simulink model "gm_uz_pmsm_model_9ph"  (R2021b)
settings: Solver=FixedStepAuto  StartTime=0.0  StopTime=0.8  RelTol=1e-3
PreLoadFcn:
  | uz_pmsm_model_9ph_init_parameter
undefined symbols (not defined in the file or in its folder): a, b, c, friction_coefficient, inertia, k_i_d, k_i_q, k_p_d, k_p_q, Kpd, L_d, L_o1, L_o2, L_q, L_x1, L_x2, L_y1, L_y2, L_zero, polepair, psi_pm, R_1, static_friction_torque, Tnd
libraries: hdlmdlgenlib x190, hdlsllib x90, dspsigops x17, simulink x3, slpidlib x2, spsAlphaBetaZerotodq0Lib x1, pid_lib x1, spsdq0toAlphaBetaZeroLib x1
(part 1 of 6)
settings Model: Creator=ts  LastModifiedBy=valen
settings SolverCC: AlgebraicLoopSolver=TrustRegion  AutoInsertRateTranBlk=on
settings DataIOCC: LimitDataPoints=on  SaveOutput=off  SaveTime=off
settings OptimizationCC: BlockReduction=off  ConditionallyExecuteInputs=off  DefaultParameterBehavior=Inlined  LifeSpan=inf
settings DebuggingCC: AlgebraicLoopMsg=error  ArtificialAlgebraicLoopMsg=none  InheritedTsInSrcMsg=none  SingleTaskRateTransMsg=error  AllowSymbolicDim=off  StrictBusMsg=ErrorOnBusTreatedAsVector  SFUnexpectedBacktrackingDiag=warning  SFNoUnconditionalDefaultTransitionDiag=warning  SFExecutionAtInitializationDiag=none  SFMachineParentedDataDiag=warning  ArithmeticOperatorsInVariantConditions=warning
settings HardwareCC: ProdBitPerPointer=32  ProdBitPerSizeT=32  ProdBitPerPtrDiffT=32  ProdLargestAtomicFloat=None  ProdIntDivRoundTo=Undefined  ProdEndianess=Unspecified  ProdWordSize=32  ProdHWDeviceType=ASIC/FPGA->ASIC/FPGA  ProdEqTarget=off
settings SFSimCC: SimUseLocalCustomCode=off  CustomCodeUndefinedFunction=UseInterfaceOnly
settings RTWCC: RTWUseLocalCustomCode=off
settings CodeAppCC: StateflowObjectComments=on
settings GRTTargetCC: TargetLangStandard=C89/C90 (ANSI)
settings ConfigComp: CovScope=ReferencedModels  CovMetricSettings=dw  CovSaveCumulativeToWorkspaceVar=on  CovSaveSingleToWorkspaceVar=on  CovExternalEMLEnable=off  CovSFcnEnable=off

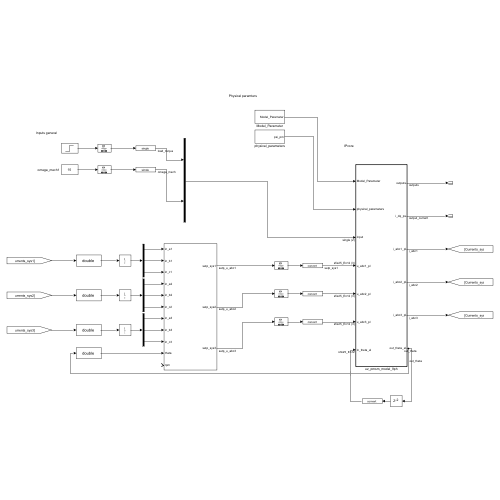
[thumbnail: Simulink's stored preview of the top-level diagram]
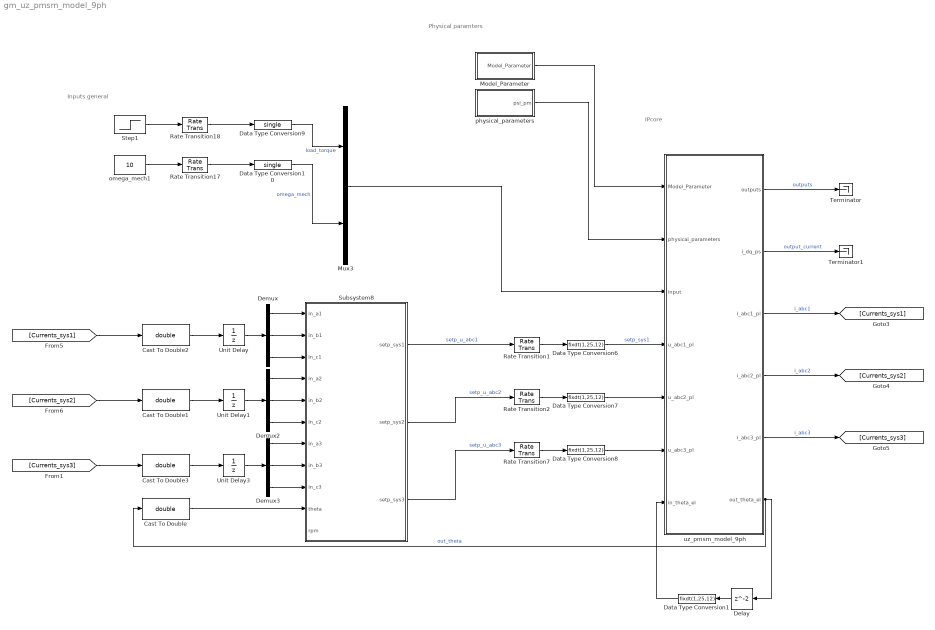
== system gm_uz_pmsm_model_9ph ==
  note: Inputs general
  note: Physical paramters
  note: IPcore
  Cast To Double{,1..3} (4 alike) : DataTypeConversion  OutDataTypeStr=double
  Data Type Conversion{1,6..8} (4 alike) : DataTypeConversion  OutDataTypeStr=fixdt(1,25,12)  RndMeth=Nearest
  Data Type Conversion10 : DataTypeConversion  OutDataTypeStr=single  RndMeth=Nearest
  Data Type Conversion9 : DataTypeConversion  OutDataTypeStr=single  RndMeth=Nearest
  Delay : Delay
  Demux : Demux  Outputs=3
  Demux2 : Demux  Outputs=3
  Demux3 : Demux  Outputs=3
  Model_Parameter : Subsystem
  Mux3 : Mux  Inputs=2
  Rate Transition{1..2,7,17..18} (5 alike) : RateTransition  OutPortSampleTime=ts
  Step1 : Step  Time=0.25  After=20  SampleTime=0
  Subsystem8 : Subsystem
  Terminator : Terminator
  Terminator1 : Terminator
  Unit Delay : UnitDelay  SampleTime=-1  HasFrameUpgradeWarning=on
  Unit Delay1 : UnitDelay  SampleTime=-1  HasFrameUpgradeWarning=on
  Unit Delay3 : UnitDelay  SampleTime=-1  HasFrameUpgradeWarning=on
  omega_mech1 : Constant  Value=10
  physical_parameters : Subsystem
  uz_pmsm_model_9ph : Subsystem  TreatAsAtomicUnit=on
  wires:
  Rate Transition7/1 -> Data Type Conversion8/1
  Rate Transition2/1 -> Data Type Conversion7/1
  Rate Transition1/1 -> Data Type Conversion6/1
  Cast To Double3/1 -> Unit Delay3/1
  Cast To Double2/1 -> Unit Delay/1
  Cast To Double1/1 -> Unit Delay1/1
  Cast To Double/1 -> Subsystem8/10(theta)
  Demux2/3 -> Subsystem8/6(in_c2)
  Demux2/2 -> Subsystem8/5(in_b2)
  Demux/1 -> Subsystem8/1(in_a1)
  Demux3/1 -> Subsystem8/7(in_a3)
  [Currents_sys3] -> Cast To Double3/1
  Unit Delay/1 -> Demux/1
  Demux3/3 -> Subsystem8/9(in_c3)
  [Currents_sys2] -> Cast To Double1/1
  [Currents_sys1] -> Cast To Double2/1
  Demux/3 -> Subsystem8/3(in_c1)
  Unit Delay1/1 -> Demux2/1
  Demux3/2 -> Subsystem8/8(in_b3)
  Demux2/1 -> Subsystem8/4(in_a2)
  Demux/2 -> Subsystem8/2(in_b1)
  Unit Delay3/1 -> Demux3/1
  Data Type Conversion7/1 -> uz_pmsm_model_9ph/5(u_abc2_pl)
  Data Type Conversion8/1 -> uz_pmsm_model_9ph/6(u_abc3_pl)
  Subsystem8/3(setp_sys3) -> Rate Transition7/1  "setp_u_abc3"
  Subsystem8/2(setp_sys2) -> Rate Transition2/1  "setp_u_abc2"
  Data Type Conversion6/1 -> uz_pmsm_model_9ph/4(u_abc1_pl)  "setp_sys1"
  Subsystem8/1(setp_sys1) -> Rate Transition1/1  "setp_u_abc1"
  Delay/1 -> Data Type Conversion1/1
  uz_pmsm_model_9ph/6(out_theta_el) -> Cast To Double/1, Delay/1  "out_theta"
  uz_pmsm_model_9ph/4(i_abc2_pl) -> [Currents_sys2]  "i_abc2"
  uz_pmsm_model_9ph/5(i_abc3_pl) -> [Currents_sys3]  "i_abc3"
  uz_pmsm_model_9ph/3(i_abc1_pl) -> [Currents_sys1]  "i_abc1"
  uz_pmsm_model_9ph/2(i_dq_ps) -> Terminator1/1  "output_current"
  Data Type Conversion1/1 -> uz_pmsm_model_9ph/7(in_theta_el)
  Mux3/1 -> uz_pmsm_model_9ph/3(input)
  Data Type Conversion9/1 -> Mux3/1  "load_torque"
  Rate Transition17/1 -> Data Type Conversion10/1
  Data Type Conversion10/1 -> Mux3/2  "omega_mech"
  Step1/1 -> Rate Transition18/1
  Rate Transition18/1 -> Data Type Conversion9/1
  omega_mech1/1 -> Rate Transition17/1
  Model_Parameter/1(Model_Parameter) -> uz_pmsm_model_9ph/1(Model_Parameter)
  uz_pmsm_model_9ph/1(outputs) -> Terminator/1  "outputs"
  physical_parameters/1(psi_pm) -> uz_pmsm_model_9ph/2(physical_parameters)

== system gm_uz_pmsm_model_9ph/Model_Parameter ==
  note: This flag determines if omega_mech is used as an input value or
      | if the mechanical system is simulated by the model
  Bus Creator : BusCreator  Inputs=4
  Constant3 : Constant  Value=0
  Data Type Conversion{3..4,9..10} (4 alike) : DataTypeConversion  OutDataTypeStr=boolean
  Rate Transition{6,8,17..18} (4 alike) : RateTransition  OutPortSampleTime=ts
  simulate_mechanical : Constant  Value=false
  simulate_mechanical1 : Constant  Value=false
  simulate_mechanical2 : Constant  Value=false
  Model_Parameter : Outport
  wires:
  Data Type Conversion3/1 -> Bus Creator/1  "reset_integrators"
  Bus Creator/1 -> Model_Parameter/1
  Data Type Conversion4/1 -> Bus Creator/2  "simulate_mechanical"
  Data Type Conversion9/1 -> Bus Creator/3  "switch_pspl"
  Data Type Conversion10/1 -> Bus Creator/4  "control_dq_abc"
  Rate Transition18/1 -> Data Type Conversion10/1
  Rate Transition17/1 -> Data Type Conversion9/1
  simulate_mechanical1/1 -> Rate Transition17/1
  Constant3/1 -> Rate Transition6/1
  Rate Transition6/1 -> Data Type Conversion3/1
  Rate Transition8/1 -> Data Type Conversion4/1
  simulate_mechanical/1 -> Rate Transition8/1
  simulate_mechanical2/1 -> Rate Transition18/1

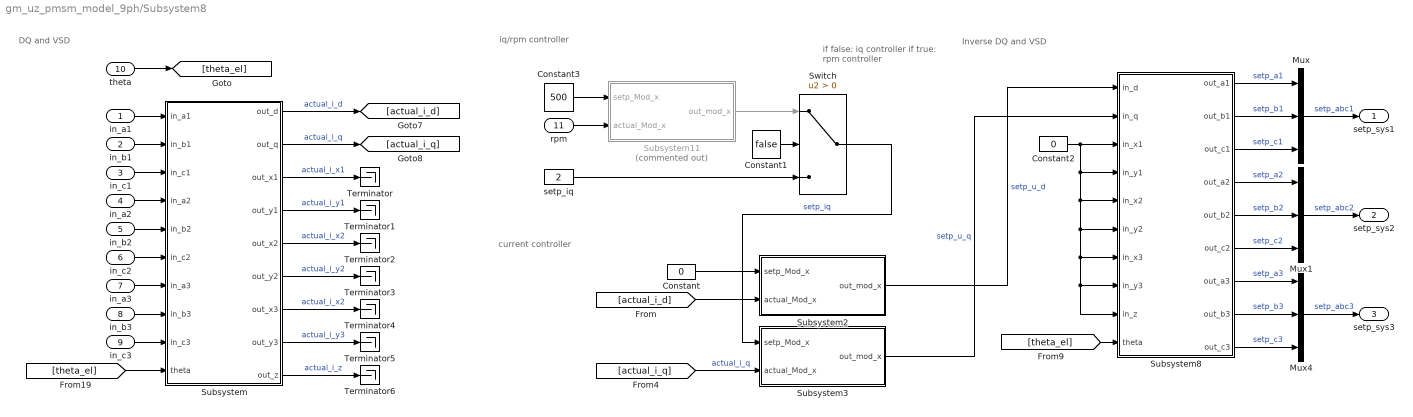
== system gm_uz_pmsm_model_9ph/Subsystem8 ==
  note: Inverse DQ and VSD
  note: if false: iq controller
      | if true: rpm controller
  note: iq/rpm controller
  note: current controller
  note: DQ and VSD
  in_a1 : Inport
  in_b1 : Inport  Port=2
  in_c1 : Inport  Port=3
  in_a2 : Inport  Port=4
  in_b2 : Inport  Port=5
  in_c2 : Inport  Port=6
  in_a3 : Inport  Port=7
  in_b3 : Inport  Port=8
  in_c3 : Inport  Port=9
  theta : Inport  Port=10
  rpm : Inport  Port=11
  Constant : Constant  Value=0
  Constant1 : Constant  Value=false
  Constant2 : Constant  Value=0
  Constant3 : Constant  Value=500
  Mux : Mux  Inputs=3
  Mux1 : Mux  Inputs=3
  Mux4 : Mux  Inputs=3
  Subsystem : Subsystem
  Subsystem11 : Subsystem  Commented=on
  Subsystem2 : Subsystem
  Subsystem3 : Subsystem
  Subsystem8 : Subsystem
  Switch : Switch  Criteria=u2 > Threshold
  Terminator{,1..6} (7 alike) : Terminator
  setp_iq : Constant  Value=2
  setp_sys1 : Outport
  setp_sys2 : Outport  Port=2
  setp_sys3 : Outport  Port=3
  wires:
  Subsystem2/1(out_mod_x) -> Subsystem8/1(in_d)  "setp_u_d"
  Subsystem3/1(out_mod_x) -> Subsystem8/2(in_q)  "setp_u_q"
  Constant3/1 -> Subsystem11/1(setp_Mod_x)
  setp_iq/1 -> Switch/3
  Constant1/1 -> Switch/2
  Switch/1 -> Subsystem3/1(setp_Mod_x)  "setp_iq"
  Subsystem11/1(out_mod_x) -> Switch/1
  Constant2/1 -> Subsystem8/4(in_y1), Subsystem8/5(in_x2), Subsystem8/6(in_y2), Subsystem8/7(in_x3), Subsystem8/9(in_z), Subsystem8/8(in_y3), Subsystem8/3(in_x1)
  [theta_el] -> Subsystem/10(theta)
  Subsystem/2(out_q) -> [actual_i_q]  "actual_i_q"
  Subsystem/1(out_d) -> [actual_i_d]  "actual_i_d"
  rpm/1 -> Subsystem11/2(actual_Mod_x)
  Subsystem8/9(out_c3) -> Mux4/3  "setp_c3"
  Subsystem8/8(out_b3) -> Mux4/2  "setp_b3"
  Subsystem8/7(out_a3) -> Mux4/1  "setp_a3"
  Mux4/1 -> setp_sys3/1  "setp_abc3"
  Subsystem8/4(out_a2) -> Mux1/1  "setp_a2"
  Subsystem8/5(out_b2) -> Mux1/2  "setp_b2"
  Subsystem8/6(out_c2) -> Mux1/3  "setp_c2"
  Mux1/1 -> setp_sys2/1  "setp_abc2"
  in_a3/1 -> Subsystem/7(in_a3)
  in_b3/1 -> Subsystem/8(in_b3)
  in_c3/1 -> Subsystem/9(in_c3)
  Subsystem/9(out_z) -> Terminator6/1  "actual_i_z"
  Subsystem/7(out_x3) -> Terminator4/1  "actual_i_x2"
  Subsystem/8(out_y3) -> Terminator5/1  "actual_i_y3"
  Mux/1 -> setp_sys1/1  "setp_abc1"
  theta/1 -> [theta_el]
  in_c2/1 -> Subsystem/6(in_c2)
  in_a2/1 -> Subsystem/4(in_a2)
  in_b2/1 -> Subsystem/5(in_b2)
  [actual_i_q] -> Subsystem3/2(actual_Mod_x)  "actual_i_q"
  in_a1/1 -> Subsystem/1(in_a1)
  Subsystem/5(out_x2) -> Terminator2/1  "actual_i_x2"
  Subsystem/6(out_y2) -> Terminator3/1  "actual_i_y2"
  Constant/1 -> Subsystem2/1(setp_Mod_x)
  [actual_i_d] -> Subsystem2/2(actual_Mod_x)
  in_c1/1 -> Subsystem/3(in_c1)
  Subsystem/3(out_x1) -> Terminator/1  "actual_i_x1"
  Subsystem8/3(out_c1) -> Mux/3  "setp_c1"
  Subsystem8/2(out_b1) -> Mux/2  "setp_b1"
  [theta_el] -> Subsystem8/10(theta)
  in_b1/1 -> Subsystem/2(in_b1)
  Subsystem8/1(out_a1) -> Mux/1  "setp_a1"
  Subsystem/4(out_y1) -> Terminator1/1  "actual_i_y1"

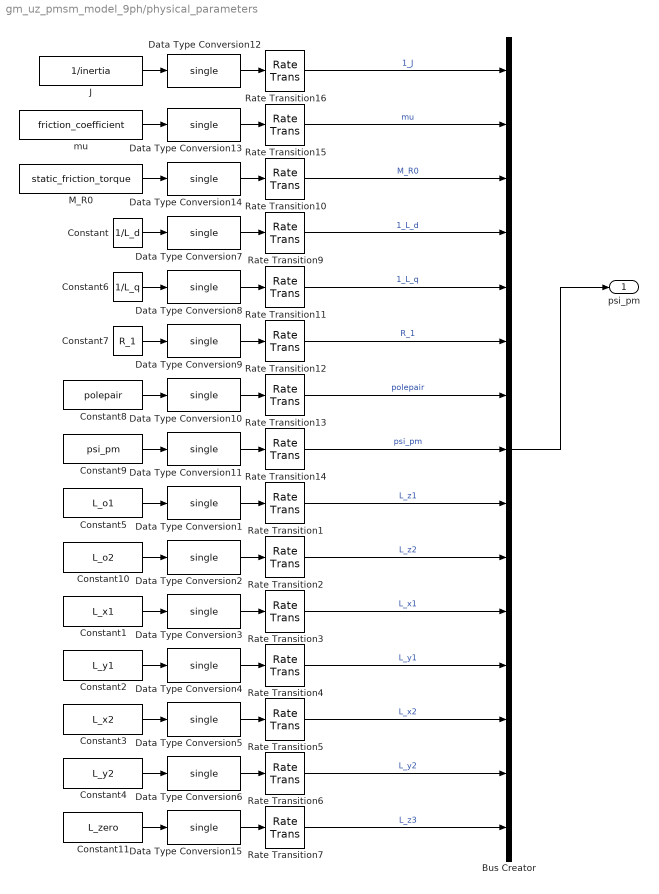
== system gm_uz_pmsm_model_9ph/physical_parameters ==
  Bus Creator : BusCreator  Inputs=15
  Constant : Constant  Value=1/L_d
  Constant1 : Constant  Value=L_x1
  Constant10 : Constant  Value=L_o2
  Constant11 : Constant  Value=L_zero
  Constant2 : Constant  Value=L_y1
  Constant3 : Constant  Value=L_x2
  Constant4 : Constant  Value=L_y2
  Constant5 : Constant  Value=L_o1
  Constant6 : Constant  Value=1/L_q
  Constant7 : Constant  Value=R_1
  Constant8 : Constant  Value=polepair
  Constant9 : Constant  Value=psi_pm
  Data Type Conversion{1..15} (15 alike) : DataTypeConversion  OutDataTypeStr=single
  J : Constant  Value=1/inertia
  M_R0 : Constant  Value=static_friction_torque
  Rate Transition{1..7,9..16} (15 alike) : RateTransition  OutPortSampleTime=ts
  mu : Constant  Value=friction_coefficient
  psi_pm : Outport
  wires:
  Constant10/1 -> Data Type Conversion2/1
  Constant5/1 -> Data Type Conversion1/1
  Constant1/1 -> Data Type Conversion3/1
  Constant2/1 -> Data Type Conversion4/1
  Constant3/1 -> Data Type Conversion5/1
  Constant4/1 -> Data Type Conversion6/1
  Rate Transition2/1 -> Bus Creator/10  "L_z2"
  Rate Transition3/1 -> Bus Creator/11  "L_x1"
  Rate Transition4/1 -> Bus Creator/12  "L_y1"
  Rate Transition5/1 -> Bus Creator/13  "L_x2"
  Rate Transition6/1 -> Bus Creator/14  "L_y2"
  Rate Transition7/1 -> Bus Creator/15  "L_z3"
  Rate Transition1/1 -> Bus Creator/9  "L_z1"
  Data Type Conversion15/1 -> Rate Transition7/1
  Constant11/1 -> Data Type Conversion15/1
  Data Type Conversion6/1 -> Rate Transition6/1
  Data Type Conversion5/1 -> Rate Transition5/1
  Data Type Conversion4/1 -> Rate Transition4/1
  Data Type Conversion3/1 -> Rate Transition3/1
  Data Type Conversion2/1 -> Rate Transition2/1
  Data Type Conversion1/1 -> Rate Transition1/1
  Constant/1 -> Data Type Conversion7/1
  Constant9/1 -> Data Type Conversion11/1
  Constant7/1 -> Data Type Conversion9/1
  Data Type Conversion13/1 -> Rate Transition15/1
  Rate Transition11/1 -> Bus Creator/5  "1_L_q"
  M_R0/1 -> Data Type Conversion14/1
  mu/1 -> Data Type Conversion13/1
  Data Type Conversion10/1 -> Rate Transition13/1
  Data Type Conversion8/1 -> Rate Transition11/1
  J/1 -> Data Type Conversion12/1
  Rate Transition9/1 -> Bus Creator/4  "1_L_d"
  Constant6/1 -> Data Type Conversion8/1
  Rate Transition15/1 -> Bus Creator/2  "mu"
  Data Type Conversion9/1 -> Rate Transition12/1
  Constant8/1 -> Data Type Conversion10/1
  Data Type Conversion11/1 -> Rate Transition14/1
  Bus Creator/1 -> psi_pm/1
  Rate Transition13/1 -> Bus Creator/7  "polepair"
  Rate Transition16/1 -> Bus Creator/1  "1_J"
  Rate Transition12/1 -> Bus Creator/6  "R_1"
  Data Type Conversion14/1 -> Rate Transition10/1
  Rate Transition14/1 -> Bus Creator/8  "psi_pm"
  Rate Transition10/1 -> Bus Creator/3  "M_R0"
  Data Type Conversion7/1 -> Rate Transition9/1
  Data Type Conversion12/1 -> Rate Transition16/1
